simulink library "lib"  (R2021a)
settings: Solver=VariableStepAuto  StartTime=0.0  StopTime=10.0  RelTol=1e-3
values from neighbouring files (symbols this model uses):
  I = [I_x;I_y;I_z]    [DATA.m]
  I_inv = inv(I_matrix)    [DATA.m]
  I_matrix = diag(I)    [DATA.m]
  I_x = 91.6*1e-2    (= 0.916)    [DATA.m]
  I_y = 25.1*1e-2    (= 0.251)    [DATA.m]
  I_z = 100.9*1e-2    (= 1.009)    [DATA.m]
  om0 = deg2rad([10, -15, 5]')    [DATA.m]
  phi0_312 = -atan(A_313_0(2,1)/A_313_0(2,2))    [DATA.m]
  phi0_313 = deg2rad(9.7)    [DATA.m]
  psi0_312 = -atan(A_313_0(1,3)/A_313_0(3,3))    [DATA.m]
  psi0_313 = deg2rad(6)    [DATA.m]
  th0_312 = asin(A_313_0(2,3))    [DATA.m]
  th0_313 = deg2rad(19)    [DATA.m]
undefined symbols (not defined in the file or in its folder): dcm0, e, i, I_f, I_r, om0_f, om0_r, om0_x, om0_y, om0_z, orbit
libraries: $bdroot x8, vrlib x1
settings Model: Creator=dvd33  LastModifiedBy=dvd33
settings SolverCC: AlgebraicLoopSolver=TrustRegion
settings DebuggingCC: SFMachineParentedDataDiag=warning

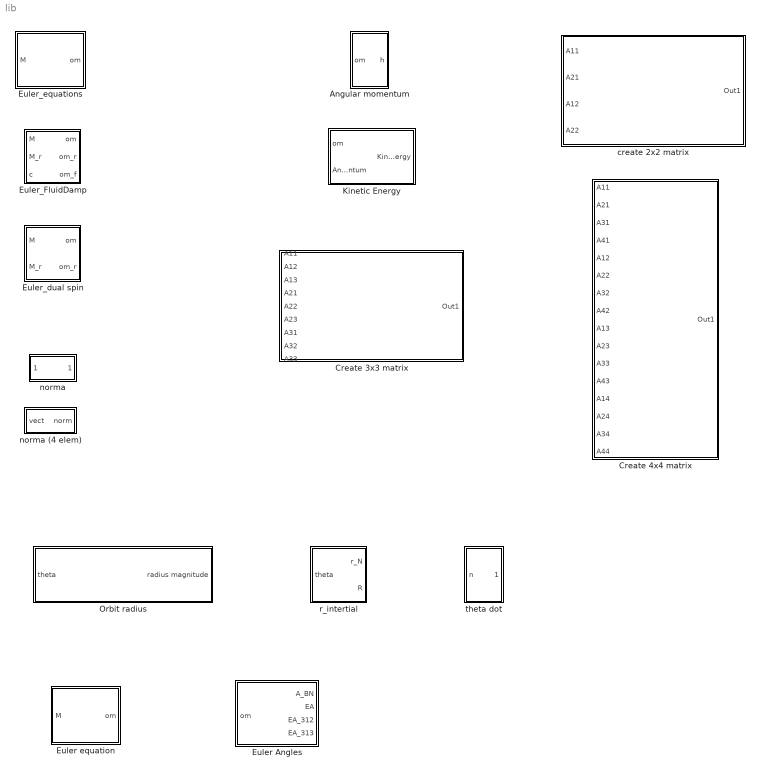
== system lib ==
  Angular momentum : Subsystem
  Create 3x3 matrix : Subsystem
  Create 4x4 matrix : Subsystem
  Euler Angles : Subsystem
  Euler equation : Subsystem
  Euler_FluidDamp : Subsystem
  Euler_dual spin : Subsystem
  Euler_equations : Subsystem
  Kinetic Energy : Subsystem
  Orbit radius : Subsystem
  create 2x2 matrix : Subsystem
  norma : Subsystem
  norma (4 elem) : Subsystem
  r_intertial : Subsystem
  theta dot : Subsystem

== system lib/Angular momentum ==
  om : Inport
  Demux : Demux  Outputs=3
  Gain : Gain  Gain=I_x
  Gain1 : Gain  Gain=I_y
  Gain2 : Gain  Gain=I_z
  Mux : Mux  Inputs=3
  h : Outport
  wires:
  Gain/1 -> Mux/1
  Demux/2 -> Gain1/1
  Gain1/1 -> Mux/2
  om/1 -> Demux/1
  Demux/3 -> Gain2/1
  Demux/1 -> Gain/1
  Mux/1 -> h/1  "Angular momentum"
  Gain2/1 -> Mux/3

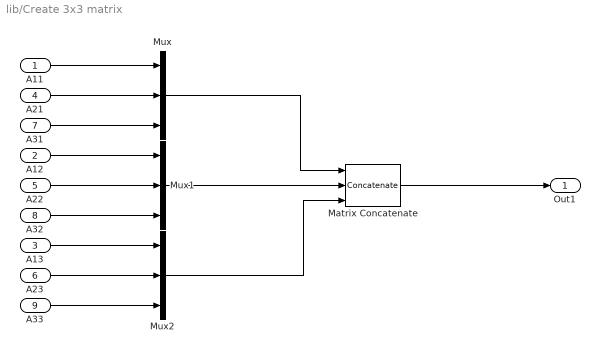
== system lib/Create 3x3 matrix ==
  A11 : Inport
  A12 : Inport  Port=2
  A13 : Inport  Port=3
  A21 : Inport  Port=4
  A22 : Inport  Port=5
  A23 : Inport  Port=6
  A31 : Inport  Port=7
  A32 : Inport  Port=8
  A33 : Inport  Port=9
  Matrix Concatenate : Concatenate  NumInputs=3  Mode=Multidimensional array  ConcatenateDimension=2
  Mux : Mux  Inputs=3
  Mux1 : Mux  Inputs=3
  Mux2 : Mux  Inputs=3
  Out1 : Outport
  wires:
  A33/1 -> Mux2/3
  A23/1 -> Mux2/2
  A13/1 -> Mux2/1
  A32/1 -> Mux1/3
  A22/1 -> Mux1/2
  A12/1 -> Mux1/1
  A21/1 -> Mux/2
  A31/1 -> Mux/3
  A11/1 -> Mux/1
  Mux2/1 -> Matrix Concatenate/3
  Mux1/1 -> Matrix Concatenate/2
  Mux/1 -> Matrix Concatenate/1
  Matrix Concatenate/1 -> Out1/1

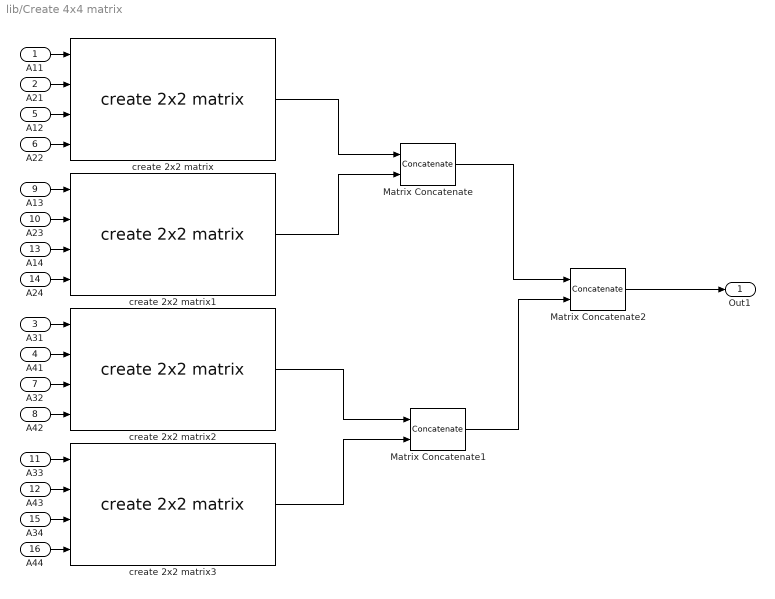
== system lib/Create 4x4 matrix ==
  A11 : Inport
  A21 : Inport  Port=2
  A31 : Inport  Port=3
  A41 : Inport  Port=4
  A12 : Inport  Port=5
  A22 : Inport  Port=6
  A32 : Inport  Port=7
  A42 : Inport  Port=8
  A13 : Inport  Port=9
  A23 : Inport  Port=10
  A33 : Inport  Port=11
  A43 : Inport  Port=12
  A14 : Inport  Port=13
  A24 : Inport  Port=14
  A34 : Inport  Port=15
  A44 : Inport  Port=16
  Matrix Concatenate : Concatenate  Mode=Multidimensional array
  Matrix Concatenate1 : Concatenate  Mode=Multidimensional array
  Matrix Concatenate2 : Concatenate  Mode=Multidimensional array  ConcatenateDimension=2
  create 2x2 matrix{,1..3} (4 alike) : $bdroot/create 2x2 matrix  SystemSampleTime=-1  Latency=0  AutoFrameSizeCalculation=off
  Out1 : Outport
  wires:
  A24/1 -> create 2x2 matrix1/4
  Matrix Concatenate1/1 -> Matrix Concatenate2/2
  create 2x2 matrix1/1 -> Matrix Concatenate/2
  Matrix Concatenate/1 -> Matrix Concatenate2/1
  create 2x2 matrix/1 -> Matrix Concatenate/1
  create 2x2 matrix2/1 -> Matrix Concatenate1/1
  A14/1 -> create 2x2 matrix1/3
  create 2x2 matrix3/1 -> Matrix Concatenate1/2
  A43/1 -> create 2x2 matrix3/2
  Matrix Concatenate2/1 -> Out1/1
  A34/1 -> create 2x2 matrix3/3
  A33/1 -> create 2x2 matrix3/1
  A44/1 -> create 2x2 matrix3/4
  A23/1 -> create 2x2 matrix1/2
  A32/1 -> create 2x2 matrix2/3
  A13/1 -> create 2x2 matrix1/1
  A21/1 -> create 2x2 matrix/2
  A12/1 -> create 2x2 matrix/3
  A42/1 -> create 2x2 matrix2/4
  A22/1 -> create 2x2 matrix/4
  A31/1 -> create 2x2 matrix2/1
  A11/1 -> create 2x2 matrix/1
  A41/1 -> create 2x2 matrix2/2

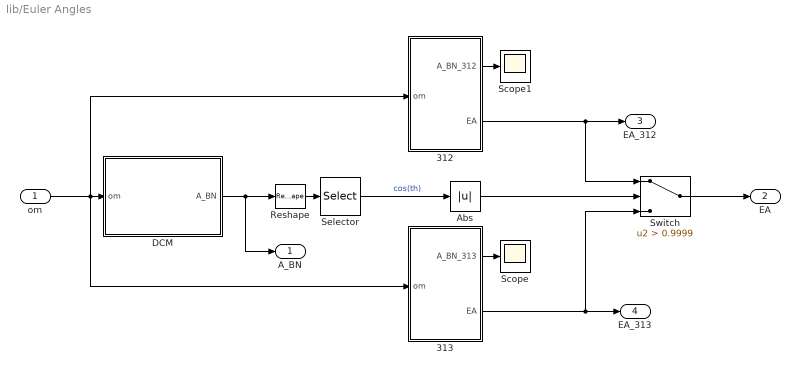
== system lib/Euler Angles ==
  om : Inport
  312 : Subsystem  TreatAsAtomicUnit=on
  313 : Subsystem  TreatAsAtomicUnit=on
  Abs : Abs
  DCM : Subsystem
  Reshape : Reshape
  Scope : Scope
  Scope1 : Scope
  Selector : Selector  InputPortWidth=9  IndexOptions=Index vector (dialog)  Indices=[9]  OutputSizes=1
  Switch : Switch  Criteria=u2 > Threshold  Threshold=0.9999
  A_BN : Outport
  EA : Outport  Port=2
  EA_312 : Outport  Port=3
  EA_313 : Outport  Port=4
  wires:
  om/1 -> 312/1(om), 313/1(om), DCM/1(om)
  DCM/1(A_BN) -> A_BN/1, Reshape/1
  Reshape/1 -> Selector/1
  Selector/1 -> Abs/1  "cos(th)"
  Abs/1 -> Switch/2
  313/1(A_BN_313) -> Scope/1
  312/1(A_BN_312) -> Scope1/1
  312/2(EA) -> EA_312/1, Switch/1
  313/2(EA) -> EA_313/1, Switch/3
  Switch/1 -> EA/1

== system lib/Euler equation ==
  M : Inport
  Cross Product : vrlib/Utilities/Cross Product
  Gain : Gain  Gain=I_matrix  Multiplication=Matrix(K*u) (u vector)
  Gain1 : Gain  Gain=I_inv  Multiplication=Matrix(K*u) (u vector)
  Integrator : Integrator  InitialCondition=om0
  Sum : Sum
  om : Outport
  wires:
  Gain/1 -> Cross Product/1
  Cross Product/1 -> Sum/1
  M/1 -> Sum/2
  Sum/1 -> Gain1/1
  Gain1/1 -> Integrator/1
  Integrator/1 -> Gain/1, Cross Product/2, om/1

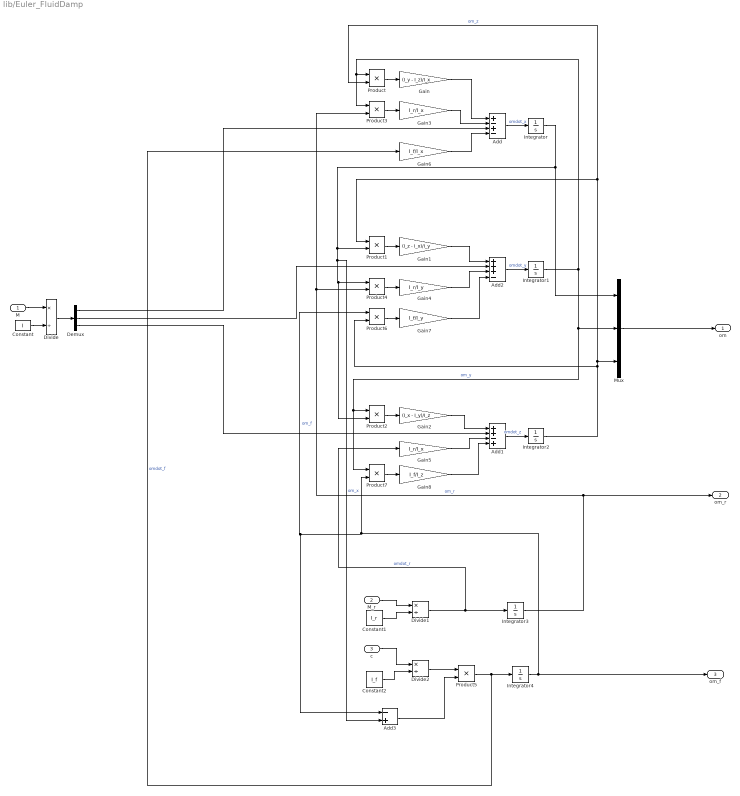
== system lib/Euler_FluidDamp ==
  M : Inport
  M_r : Inport  Port=2
  c : Inport  Port=3
  Add : Sum  Inputs=+-+-
  Add1 : Sum  Inputs=++-+
  Add2 : Sum  Inputs=+++-
  Add3 : Sum  Inputs=-+
  Constant : Constant  Value=I
  Constant1 : Constant  Value=I_r
  Constant2 : Constant  Value=I_f
  Demux : Demux  Outputs=3
  Divide : Product  Inputs=*/
  Divide1 : Product  Inputs=*/
  Divide2 : Product  Inputs=*/
  Gain : Gain  Gain=(I_y - I_z)/I_x
  Gain1 : Gain  Gain=(I_z - I_x)/I_y
  Gain2 : Gain  Gain=(I_x - I_y)/I_z
  Gain3 : Gain  Gain=I_r/I_x
  Gain4 : Gain  Gain=I_r/I_y
  Gain5 : Gain  Gain=I_r/I_x
  Gain6 : Gain  Gain=I_f/I_x
  Gain7 : Gain  Gain=I_f/I_y
  Gain8 : Gain  Gain=I_f/I_z
  Integrator : Integrator  InitialCondition=om0_x
  Integrator1 : Integrator  InitialCondition=om0_y
  Integrator2 : Integrator  InitialCondition=om0_z
  Integrator3 : Integrator  InitialCondition=om0_r
  Integrator4 : Integrator  InitialCondition=om0_f
  Mux : Mux  Inputs=3
  Product{,1..7} (8 alike) : Product
  om : Outport
  om_r : Outport  Port=2
  om_f : Outport  Port=3
  wires:
  Add3/1 -> Product5/2
  M/1 -> Divide/1
  Product5/1 -> Gain6/1, Integrator4/1  "omdot_f"
  Add/1 -> Integrator/1  "omdot_x"
  Integrator1/1 -> Product2/1, Product7/1, Mux/2, Product3/1, Product/1  "om_y"
  Integrator2/1 -> Product1/1, Product/2, Mux/3, Product6/2  "om_z"
  Product/1 -> Gain/1
  Add2/1 -> Integrator1/1  "omdot_y"
  Demux/3 -> Add1/2
  M_r/1 -> Divide1/1
  Product2/1 -> Gain2/1
  Gain7/1 -> Add2/4
  Gain8/1 -> Add1/4
  Integrator3/1 -> om_r/1, Product4/2, Product3/2  "om_r"
  Gain4/1 -> Add2/3
  Constant/1 -> Divide/2
  Product1/1 -> Gain1/1
  Integrator/1 -> Mux/1, Product2/2, Product4/1, Add3/2, Product1/2  "om_x"
  Gain1/1 -> Add2/1
  Demux/1 -> Add/3
  Constant2/1 -> Divide2/2
  Add1/1 -> Integrator2/1  "omdot_z"
  Product4/1 -> Gain4/1
  Demux/2 -> Add2/2
  c/1 -> Divide2/1
  Gain2/1 -> Add1/1
  Product6/1 -> Gain7/1
  Divide1/1 -> Gain5/1, Integrator3/1  "omdot_r"
  Divide2/1 -> Product5/1
  Gain5/1 -> Add1/3
  Product3/1 -> Gain3/1
  Constant1/1 -> Divide1/2
  Integrator4/1 -> om_f/1, Add3/1, Product6/1, Product7/2  "om_f"
  Gain6/1 -> Add/4
  Divide/1 -> Demux/1
  Gain/1 -> Add/1
  Product7/1 -> Gain8/1
  Gain3/1 -> Add/2
  Mux/1 -> om/1

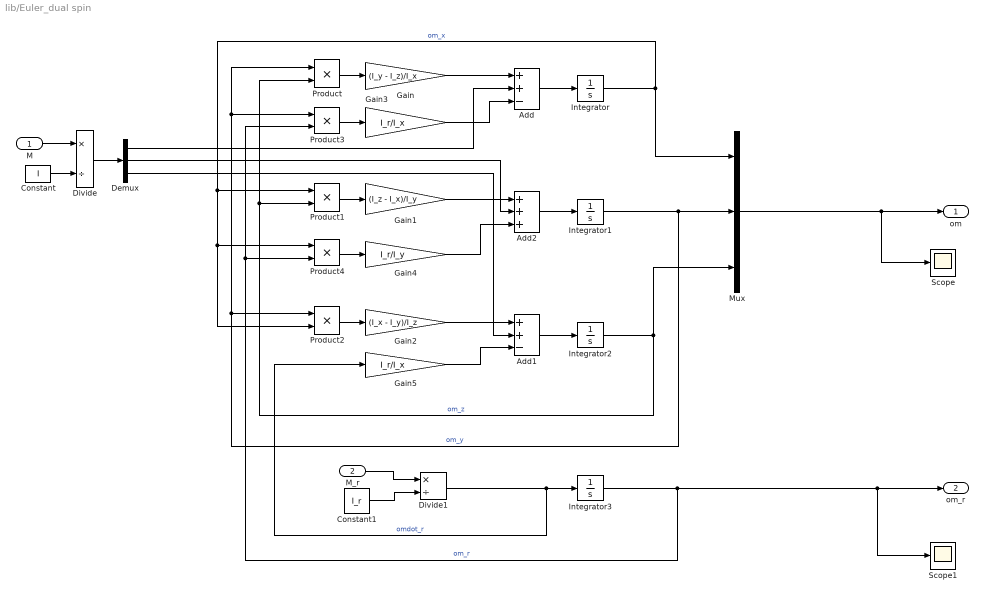
== system lib/Euler_dual spin ==
  M : Inport
  M_r : Inport  Port=2
  Add : Sum  Inputs=++-
  Add1 : Sum  Inputs=++-
  Add2 : Sum  Inputs=+++
  Constant : Constant  Value=I
  Constant1 : Constant  Value=I_r
  Demux : Demux  Outputs=3
  Divide : Product  Inputs=*/
  Divide1 : Product  Inputs=*/
  Gain : Gain  Gain=(I_y - I_z)/I_x
  Gain1 : Gain  Gain=(I_z - I_x)/I_y
  Gain2 : Gain  Gain=(I_x - I_y)/I_z
  Gain3 : Gain  Gain=I_r/I_x
  Gain4 : Gain  Gain=I_r/I_y
  Gain5 : Gain  Gain=I_r/I_x
  Integrator : Integrator  InitialCondition=om0_x
  Integrator1 : Integrator  InitialCondition=om0_y
  Integrator2 : Integrator  InitialCondition=om0_z
  Integrator3 : Integrator  InitialCondition=om0_r
  Mux : Mux  Inputs=3
  Product{,1..4} (5 alike) : Product
  Scope : Scope
  Scope1 : Scope
  om : Outport
  om_r : Outport  Port=2
  wires:
  Add2/1 -> Integrator1/1
  M_r/1 -> Divide1/1
  Product4/1 -> Gain4/1
  Gain5/1 -> Add1/3
  Demux/1 -> Add/2
  Product3/1 -> Gain3/1
  Add1/1 -> Integrator2/1
  Gain3/1 -> Add/3
  Add/1 -> Integrator/1
  Demux/3 -> Add1/2
  Integrator3/1 -> Scope1/1, om_r/1, Product3/2, Product4/2  "om_r"
  Constant1/1 -> Divide1/2
  Divide/1 -> Demux/1
  M/1 -> Divide/1
  Product2/1 -> Gain2/1
  Product/1 -> Gain/1
  Demux/2 -> Add2/2
  Divide1/1 -> Integrator3/1, Gain5/1  "omdot_r"
  Gain1/1 -> Add2/1
  Integrator/1 -> Product1/1, Product4/1, Product2/2, Mux/1  "om_x"
  Integrator2/1 -> Product/2, Product1/2, Mux/3  "om_z"
  Gain4/1 -> Add2/3
  Constant/1 -> Divide/2
  Integrator1/1 -> Mux/2, Product2/1, Product3/1, Product/1  "om_y"
  Gain/1 -> Add/1
  Gain2/1 -> Add1/1
  Product1/1 -> Gain1/1
  Mux/1 -> Scope/1, om/1

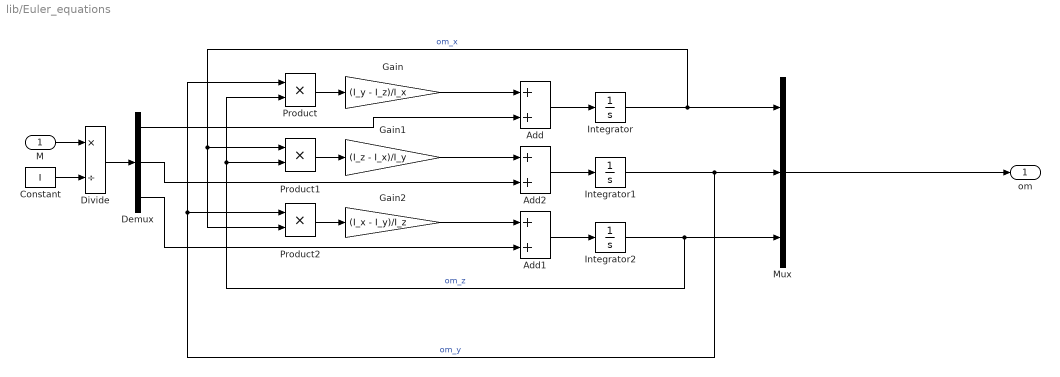
== system lib/Euler_equations ==
  M : Inport
  Add : Sum
  Add1 : Sum
  Add2 : Sum
  Constant : Constant  Value=I
  Demux : Demux  Outputs=3
  Divide : Product  Inputs=*/
  Gain : Gain  Gain=(I_y - I_z)/I_x
  Gain1 : Gain  Gain=(I_z - I_x)/I_y
  Gain2 : Gain  Gain=(I_x - I_y)/I_z
  Integrator : Integrator  InitialCondition=om0_x
  Integrator1 : Integrator  InitialCondition=om0_y
  Integrator2 : Integrator  InitialCondition=om0_z
  Mux : Mux  Inputs=3
  Product : Product
  Product1 : Product
  Product2 : Product
  om : Outport
  wires:
  Divide/1 -> Demux/1
  Product/1 -> Gain/1
  Demux/2 -> Add2/2
  Demux/1 -> Add/2
  Mux/1 -> om/1
  Gain1/1 -> Add2/1
  Gain/1 -> Add/1
  Constant/1 -> Divide/2
  Add/1 -> Integrator/1
  Demux/3 -> Add1/2
  Integrator1/1 -> Mux/2, Product/1, Product2/1  "om_y"
  Integrator/1 -> Mux/1, Product2/2, Product1/1  "om_x"
  Product1/1 -> Gain1/1
  Add2/1 -> Integrator1/1
  M/1 -> Divide/1
  Add1/1 -> Integrator2/1
  Product2/1 -> Gain2/1
  Gain2/1 -> Add1/1
  Integrator2/1 -> Mux/3, Product/2, Product1/2  "om_z"

== system lib/Kinetic Energy ==
  om : Inport
  Angular momentum : Inport  Port=2
  Dot Product : DotProduct  InputSameDT=on  OutDataTypeStr=Inherit: Inherit via internal rule
  Gain3 : Gain  Gain=0.5
  Kinectic Energy : Outport
  wires:
  Gain3/1 -> Dot Product/2
  om/1 -> Dot Product/1
  Dot Product/1 -> Kinectic Energy/1  "Kinectic Energy"
  Angular momentum/1 -> Gain3/1

== system lib/Orbit radius ==
  theta : Inport
  Add1 : Sum
  Constant : Constant  Value=orbit.a*(1-orbit.e^2)
  Constant1 : Constant
  Divide : Product  Inputs=*/
  Product : Product
  Trigonometric Function : Trigonometry  Operator=cos
  eccentricity : Constant  Value=orbit.e
  radius magnitude : Outport
  wires:
  Constant1/1 -> Add1/1
  theta/1 -> Trigonometric Function/1
  Trigonometric Function/1 -> Product/2
  Add1/1 -> Divide/2
  eccentricity/1 -> Product/1
  Divide/1 -> radius magnitude/1
  Product/1 -> Add1/2
  Constant/1 -> Divide/1

== system lib/create 2x2 matrix ==
  A11 : Inport
  A21 : Inport  Port=2
  A12 : Inport  Port=3
  A22 : Inport  Port=4
  Matrix Concatenate : Concatenate  Mode=Multidimensional array  ConcatenateDimension=2
  Mux : Mux  Inputs=2
  Mux1 : Mux  Inputs=2
  Out1 : Outport
  wires:
  Matrix Concatenate/1 -> Out1/1
  Mux/1 -> Matrix Concatenate/1
  Mux1/1 -> Matrix Concatenate/2
  A11/1 -> Mux/1
  A12/1 -> Mux/2
  A21/1 -> Mux1/1
  A22/1 -> Mux1/2

== system lib/norma ==
  vect : Inport
  Add : Sum  Inputs=+++
  Demux : Demux  Outputs=3
  Sqrt : Sqrt  SaturateOnIntegerOverflow=on
  Square : Math  Operator=square  SaturateOnIntegerOverflow=on
  Square1 : Math  Operator=square  SaturateOnIntegerOverflow=on
  Square2 : Math  Operator=square  SaturateOnIntegerOverflow=on
  norm : Outport
  wires:
  Add/1 -> Sqrt/1
  Square1/1 -> Add/2
  Square2/1 -> Add/3
  Sqrt/1 -> norm/1
  Demux/3 -> Square2/1
  Demux/2 -> Square1/1
  vect/1 -> Demux/1
  Square/1 -> Add/1
  Demux/1 -> Square/1

== system lib/norma (4 elem) ==
  vect : Inport
  Add : Sum  Inputs=++++
  Demux : Demux
  Sqrt : Sqrt  SaturateOnIntegerOverflow=on
  Square{,1..3} (4 alike) : Math  Operator=square  SaturateOnIntegerOverflow=on
  norm : Outport
  wires:
  vect/1 -> Demux/1
  Square/1 -> Add/1
  Demux/4 -> Square3/1
  Square2/1 -> Add/3
  Sqrt/1 -> norm/1
  Demux/1 -> Square/1
  Square1/1 -> Add/2
  Add/1 -> Sqrt/1
  Demux/2 -> Square1/1
  Demux/3 -> Square2/1
  Square3/1 -> Add/4

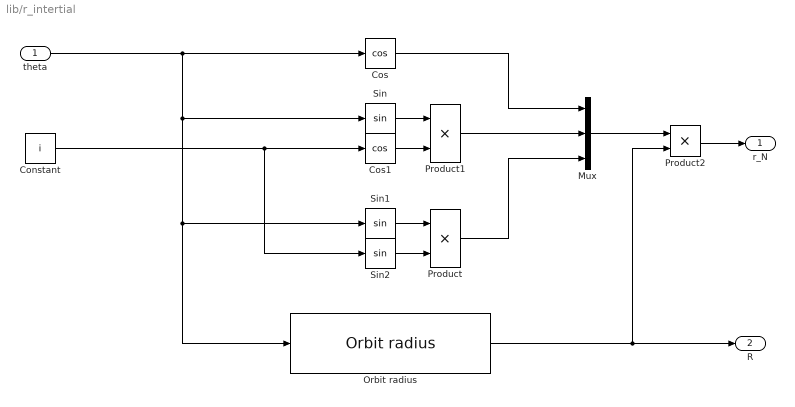
== system lib/r_intertial ==
  theta : Inport
  Constant : Constant  Value=i
  Cos : Trigonometry  Operator=cos
  Cos1 : Trigonometry  Operator=cos
  Mux : Mux  Inputs=3
  Orbit radius : $bdroot/Orbit radius  SystemSampleTime=-1  VariantActivationTime=update diagram  Latency=0  AutoFrameSizeCalculation=off
  Product : Product
  Product1 : Product
  Product2 : Product
  Sin : Trigonometry
  Sin1 : Trigonometry
  Sin2 : Trigonometry
  r_N : Outport
  R : Outport  Port=2
  wires:
  Mux/1 -> Product2/1
  Sin2/1 -> Product/2
  Orbit radius/1 -> R/1, Product2/2
  Cos/1 -> Mux/1
  Cos1/1 -> Product1/2
  Constant/1 -> Cos1/1, Sin2/1
  Product2/1 -> r_N/1
  Product/1 -> Mux/3
  theta/1 -> Sin1/1, Orbit radius/1, Sin/1, Cos/1
  Sin/1 -> Product1/1
  Product1/1 -> Mux/2
  Sin1/1 -> Product/1

== system lib/theta dot ==
  n : Inport
  Constant : Constant
  Constant1 : Constant  Value=(1-e^2)^(3/2)
  Cos : Trigonometry  Operator=cos
  Divide : Product  Inputs=*/
  Gain : Gain  Gain=e
  Integrator : Integrator
  Product : Product
  Square1 : Math  Operator=square  SaturateOnIntegerOverflow=on
  Sum1 : Sum
  theta : Outport
  wires:
  Divide/1 -> Integrator/1  "theta dot"
  Product/1 -> Divide/1
  Sum1/1 -> Square1/1
  Square1/1 -> Product/2
  Gain/1 -> Sum1/1
  Constant1/1 -> Divide/2
  Integrator/1 -> Cos/1, theta/1  "theta"
  Cos/1 -> Gain/1
  n/1 -> Product/1
  Constant/1 -> Sum1/2

== system lib/Euler Angles/312 ==
  om : Inport
  A_312 : Subsystem
  Angles 312 : Subsystem
  A_BN_312 : Outport
  EA : Outport  Port=2
  wires:
  A_312/1(A_BN_312) -> A_BN_312/1
  om/1 -> Angles 312/1(om)
  Angles 312/1(EA) -> EA/1, A_312/1(EA)

== system lib/Euler Angles/313 ==
  om : Inport
  A_313 : Subsystem
  Angles 313 : Subsystem
  Display : Display
  A_BN_313 : Outport
  EA : Outport  Port=2
  wires:
  om/1 -> Angles 313/1(om)
  A_313/1(A_BN_313) -> A_BN_313/1
  Angles 313/1(EA) -> Display/1, EA/1, A_313/1(EA)

== system lib/Euler Angles/DCM ==
  om : Inport
  Gain : Gain  Gain=-1
  Integrator : Integrator  InitialCondition=dcm0
  Matrix Multiply : Product  Multiplication=Matrix(*)
  Orthonormalization : Subsystem
  Subsystem : Subsystem
  A_BN : Outport
  wires:
  om/1 -> Subsystem/1(om)
  Subsystem/1(om^) -> Gain/1
  Gain/1 -> Matrix Multiply/1
  Matrix Multiply/1 -> Integrator/1
  Integrator/1 -> Orthonormalization/1(A0)
  Orthonormalization/1(A) -> A_BN/1, Matrix Multiply/2

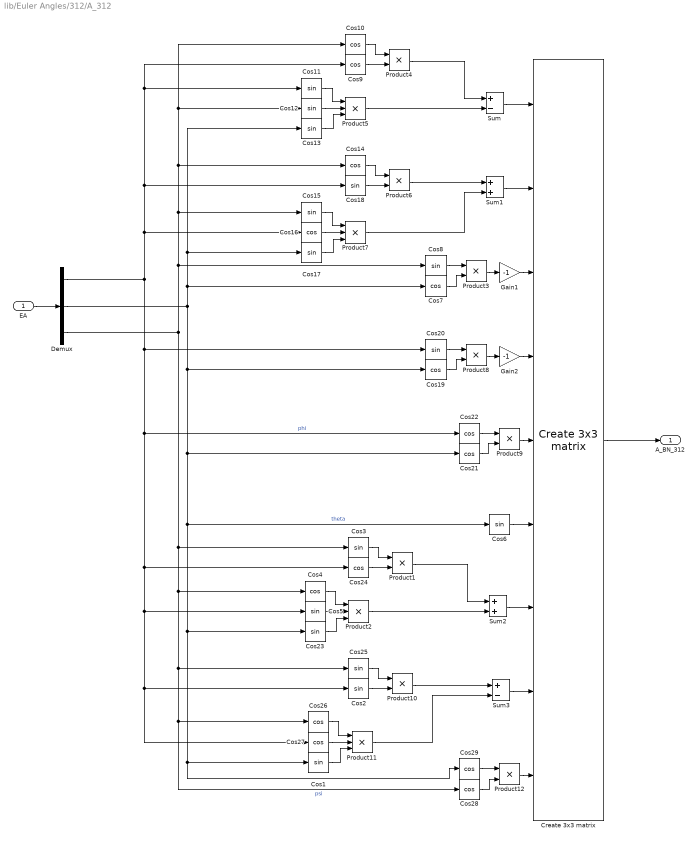
== system lib/Euler Angles/312/A_312 ==
  EA : Inport
  Cos{1..3,5..6,8,11..13,15,17..18,20,23,25} (15 alike) : Trigonometry
  Cos{4,7,9..10,14,16,19,21..22,24,26..29} (14 alike) : Trigonometry  Operator=cos
  Create 3x3 matrix : $bdroot/Create 3x3 matrix  SystemSampleTime=-1  VariantActivationTime=update diagram  Latency=0  AutoFrameSizeCalculation=off
  Demux : Demux  Outputs=3
  Gain1 : Gain  Gain=-1
  Gain2 : Gain  Gain=-1
  Product{1,3..4,6,8..10,12} (8 alike) : Product
  Product{2,5,7,11} (4 alike) : Product  Inputs=3
  Sum : Sum  Inputs=+-
  Sum1 : Sum
  Sum2 : Sum
  Sum3 : Sum  Inputs=+-
  A_BN_312 : Outport
  wires:
  Cos10/1 -> Product4/1
  Cos18/1 -> Product6/2
  Cos15/1 -> Product7/1
  Cos16/1 -> Product7/2
  Product3/1 -> Gain1/1
  Product7/1 -> Sum1/2
  Cos13/1 -> Product5/3
  Cos6/1 -> Create 3x3 matrix/6
  Cos14/1 -> Product6/1
  Cos17/1 -> Product7/3
  Cos11/1 -> Product5/1
  Product5/1 -> Sum/2
  Cos12/1 -> Product5/2
  Product4/1 -> Sum/1
  Sum1/1 -> Create 3x3 matrix/2
  Cos9/1 -> Product4/2
  Gain2/1 -> Create 3x3 matrix/4
  Cos8/1 -> Product3/1
  Cos7/1 -> Product3/2
  Sum/1 -> Create 3x3 matrix/1
  Product6/1 -> Sum1/1
  Create 3x3 matrix/1 -> A_BN_312/1
  Gain1/1 -> Create 3x3 matrix/3
  Cos19/1 -> Product8/2
  Cos20/1 -> Product8/1
  Product8/1 -> Gain2/1
  Cos21/1 -> Product9/2
  Cos22/1 -> Product9/1
  Product9/1 -> Create 3x3 matrix/5
  Sum2/1 -> Create 3x3 matrix/7
  Cos3/1 -> Product1/1
  Product1/1 -> Sum2/1
  Cos24/1 -> Product1/2
  Cos5/1 -> Product2/2
  Product2/1 -> Sum2/2
  Cos4/1 -> Product2/1
  Cos23/1 -> Product2/3
  Cos1/1 -> Product11/3
  Cos26/1 -> Product11/1
  Cos2/1 -> Product10/2
  Product10/1 -> Sum3/1
  Cos25/1 -> Product10/1
  Product11/1 -> Sum3/2
  Cos27/1 -> Product11/2
  Sum3/1 -> Create 3x3 matrix/8
  Cos28/1 -> Product12/2
  Cos29/1 -> Product12/1
  Product12/1 -> Create 3x3 matrix/9
  Demux/2 -> Cos17/1, Cos13/1, Cos7/1, Cos19/1, Cos21/1, Cos6/1, Cos23/1, Cos29/1, Cos1/1  "theta"
  Demux/3 -> Cos28/1, Cos26/1, Cos25/1, Cos4/1, Cos3/1, Cos12/1, Cos10/1, Cos14/1, Cos15/1, Cos8/1  "psi"
  Demux/1 -> Cos11/1, Cos9/1, Cos18/1, Cos16/1, Cos20/1, Cos22/1, Cos2/1, Cos27/1, Cos5/1, Cos24/1  "phi"
  EA/1 -> Demux/1

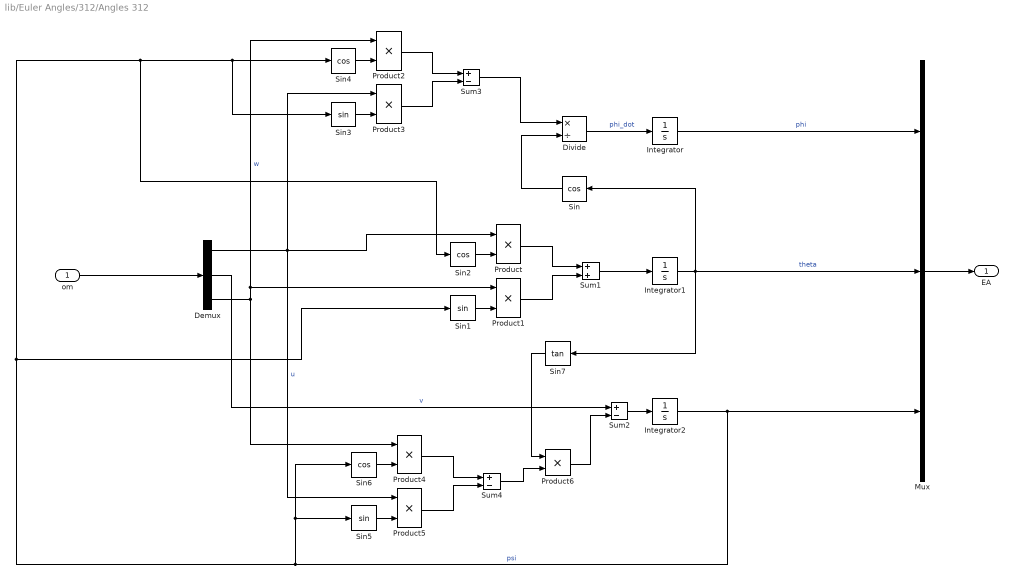
== system lib/Euler Angles/312/Angles 312 ==
  om : Inport
  Demux : Demux  Outputs=3
  Divide : Product  Inputs=*/
  Integrator : Integrator  InitialCondition=phi0_312  WrapState=on
  Integrator1 : Integrator  InitialCondition=th0_312  WrapState=on
  Integrator2 : Integrator  InitialCondition=psi0_312  WrapState=on
  Mux : Mux  Inputs=3
  Product{,1..6} (7 alike) : Product
  Sin{,2,4,6} (4 alike) : Trigonometry  Operator=cos
  Sin1 : Trigonometry
  Sin3 : Trigonometry
  Sin5 : Trigonometry
  Sin7 : Trigonometry  Operator=tan
  Sum1 : Sum
  Sum2 : Sum  Inputs=+-
  Sum3 : Sum  Inputs=+-
  Sum4 : Sum  Inputs=+-
  EA : Outport
  wires:
  Sin2/1 -> Product/2
  Sum2/1 -> Integrator2/1
  Product2/1 -> Sum3/1
  Sin7/1 -> Product6/1
  Product/1 -> Sum1/1
  Sin/1 -> Divide/2
  Demux/1 -> Product5/1, Product/1, Product3/1  "u"
  Product3/1 -> Sum3/2
  Integrator/1 -> Mux/1  "phi"
  Integrator1/1 -> Sin7/1, Mux/2, Sin/1  "theta"
  Sin6/1 -> Product4/2
  Product5/1 -> Sum4/2
  Sum3/1 -> Divide/1
  Product4/1 -> Sum4/1
  om/1 -> Demux/1
  Sin5/1 -> Product5/2
  Product6/1 -> Sum2/2
  Sum1/1 -> Integrator1/1
  Divide/1 -> Integrator/1  "phi_dot"
  Sin3/1 -> Product3/2
  Sin1/1 -> Product1/2
  Product1/1 -> Sum1/2
  Sin4/1 -> Product2/2
  Demux/3 -> Product4/1, Product1/1, Product2/1  "w"
  Integrator2/1 -> Sin1/1, Sin2/1, Sin4/1, Sin3/1, Sin5/1, Sin6/1, Mux/3  "psi"
  Demux/2 -> Sum2/1  "v"
  Sum4/1 -> Product6/2
  Mux/1 -> EA/1

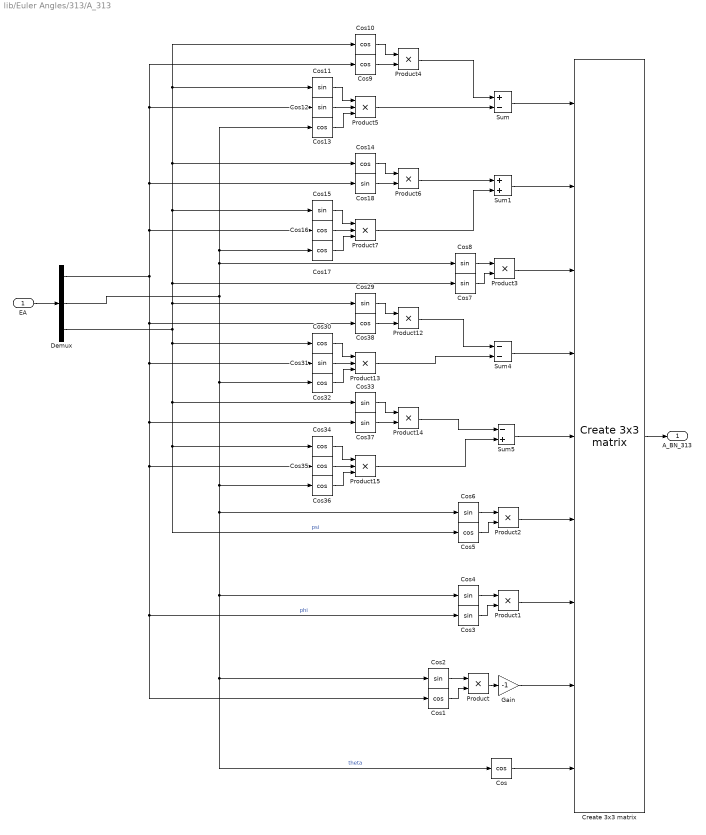
== system lib/Euler Angles/313/A_313 ==
  EA : Inport
  Cos{,1,5,9..10,13..14,16..17,30,32,34..36,38} (15 alike) : Trigonometry  Operator=cos
  Cos{2..4,6..8,11..12,15,18,29,31,33,37} (14 alike) : Trigonometry
  Create 3x3 matrix : $bdroot/Create 3x3 matrix  SystemSampleTime=-1  VariantActivationTime=update diagram  Latency=0  AutoFrameSizeCalculation=off
  Demux : Demux  Outputs=3
  Gain : Gain  Gain=-1
  Product{,1..4,6,12,14} (8 alike) : Product
  Product{5,7,13,15} (4 alike) : Product  Inputs=3
  Sum : Sum  Inputs=+-
  Sum1 : Sum
  Sum4 : Sum  Inputs=--
  Sum5 : Sum  Inputs=-+
  A_BN_313 : Outport
  wires:
  Cos1/1 -> Product/2
  Cos30/1 -> Product13/1
  Cos35/1 -> Product15/2
  Product1/1 -> Create 3x3 matrix/7
  Create 3x3 matrix/1 -> A_BN_313/1
  Product6/1 -> Sum1/1
  Cos/1 -> Create 3x3 matrix/9
  Cos31/1 -> Product13/2
  Cos34/1 -> Product15/1
  Product13/1 -> Sum4/2
  Sum/1 -> Create 3x3 matrix/1
  Cos7/1 -> Product3/2
  Cos32/1 -> Product13/3
  Cos8/1 -> Product3/1
  Sum4/1 -> Create 3x3 matrix/4
  Gain/1 -> Create 3x3 matrix/8
  Sum5/1 -> Create 3x3 matrix/5
  Cos9/1 -> Product4/2
  Sum1/1 -> Create 3x3 matrix/2
  Cos3/1 -> Product1/2
  Product4/1 -> Sum/1
  Cos2/1 -> Product/1
  Cos12/1 -> Product5/2
  Product5/1 -> Sum/2
  Product12/1 -> Sum4/1
  Cos33/1 -> Product14/1
  Cos11/1 -> Product5/1
  Cos29/1 -> Product12/1
  Cos17/1 -> Product7/3
  Product/1 -> Gain/1
  Cos37/1 -> Product14/2
  Product14/1 -> Sum5/1
  Product2/1 -> Create 3x3 matrix/6
  Cos14/1 -> Product6/1
  Cos6/1 -> Product2/1
  Cos4/1 -> Product1/1
  Cos13/1 -> Product5/3
  Product7/1 -> Sum1/2
  Product3/1 -> Create 3x3 matrix/3
  Cos38/1 -> Product12/2
  Demux/3 -> Cos33/1, Cos34/1, Cos5/1, Cos30/1, Cos11/1, Cos10/1, Cos14/1, Cos15/1, Cos7/1, Cos29/1  "psi"
  Cos5/1 -> Product2/2
  Cos16/1 -> Product7/2
  Cos36/1 -> Product15/3
  Cos15/1 -> Product7/1
  Demux/1 -> Cos16/1, Cos18/1, Cos12/1, Cos9/1, Cos31/1, Cos35/1, Cos1/1, Cos3/1, Cos37/1, Cos38/1  "phi"
  Cos18/1 -> Product6/2
  Product15/1 -> Sum5/2
  Demux/2 -> Cos13/1, Cos17/1, Cos8/1, Cos36/1, Cos2/1, Cos/1, Cos4/1, Cos6/1, Cos32/1  "theta"
  Cos10/1 -> Product4/1
  EA/1 -> Demux/1

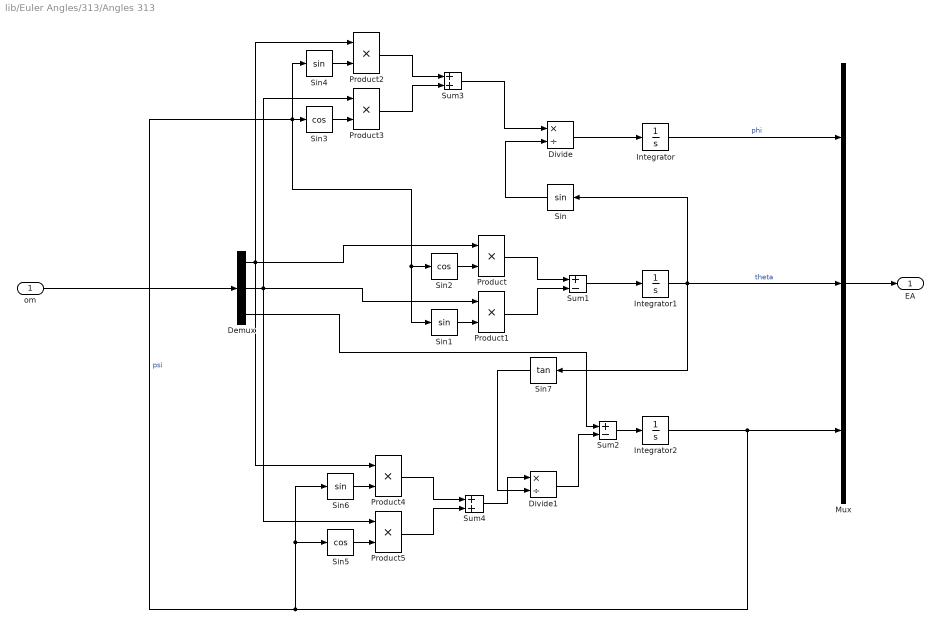
== system lib/Euler Angles/313/Angles 313 ==
  om : Inport
  Demux : Demux  Outputs=3
  Divide : Product  Inputs=*/
  Divide1 : Product  Inputs=*/
  Integrator : Integrator  InitialCondition=phi0_313  WrapState=on
  Integrator1 : Integrator  InitialCondition=th0_313  WrapState=on
  Integrator2 : Integrator  InitialCondition=psi0_313  WrapState=on
  Mux : Mux  Inputs=3
  Product{,1..5} (6 alike) : Product
  Sin{,1,4,6} (4 alike) : Trigonometry
  Sin2 : Trigonometry  Operator=cos
  Sin3 : Trigonometry  Operator=cos
  Sin5 : Trigonometry  Operator=cos
  Sin7 : Trigonometry  Operator=tan
  Sum1 : Sum  Inputs=+-
  Sum2 : Sum  Inputs=+-
  Sum3 : Sum
  Sum4 : Sum
  EA : Outport
  wires:
  Integrator2/1 -> Sin5/1, Sin6/1, Sin3/1, Sin4/1, Sin1/1, Sin2/1, Mux/3  "psi"
  Demux/3 -> Sum2/1
  Sin4/1 -> Product2/2
  Product1/1 -> Sum1/2
  Sin1/1 -> Product1/2
  Sin3/1 -> Product3/2
  Demux/2 -> Product1/1, Product5/1, Product3/1
  Divide/1 -> Integrator/1
  Sum1/1 -> Integrator1/1
  Divide1/1 -> Sum2/2
  Sin5/1 -> Product5/2
  Sum4/1 -> Divide1/1
  om/1 -> Demux/1
  Product4/1 -> Sum4/1
  Sum3/1 -> Divide/1
  Product5/1 -> Sum4/2
  Sin6/1 -> Product4/2
  Integrator/1 -> Mux/1  "phi"
  Product3/1 -> Sum3/2
  Demux/1 -> Product4/1, Product2/1, Product/1
  Sin/1 -> Divide/2
  Product/1 -> Sum1/1
  Sin7/1 -> Divide1/2
  Product2/1 -> Sum3/1
  Sum2/1 -> Integrator2/1
  Sin2/1 -> Product/2
  Mux/1 -> EA/1
  Integrator1/1 -> Sin7/1, Mux/2, Sin/1  "theta"

== system lib/Euler Angles/DCM/Orthonormalization ==
  A0 : Inport
  Gain : Gain  Gain=3/2
  Gain1 : Gain  Gain=1/2
  Matrix Multiply : Product  Inputs=3  Multiplication=Matrix(*)
  Sum : Sum  Inputs=+-
  Transpose : Math  Operator=transpose  SaturateOnIntegerOverflow=on
  A : Outport
  wires:
  Sum/1 -> A/1
  Gain/1 -> Sum/1
  A0/1 -> Matrix Multiply/1, Transpose/1, Gain1/1, Gain/1
  Transpose/1 -> Matrix Multiply/2
  Gain1/1 -> Matrix Multiply/3
  Matrix Multiply/1 -> Sum/2

== system lib/Euler Angles/DCM/Subsystem ==
  om : Inport
  Constant : Constant  Value=0
  Create 3x3 matrix : $bdroot/Create 3x3 matrix  SystemSampleTime=-1  VariantActivationTime=update diagram  Latency=0  AutoFrameSizeCalculation=off
  Demux : Demux  Outputs=3
  Gain : Gain  Gain=-1
  Gain1 : Gain  Gain=-1
  Gain2 : Gain  Gain=-1
  om^ : Outport
  wires:
  Create 3x3 matrix/1 -> om^/1
  Constant/1 -> Create 3x3 matrix/9, Create 3x3 matrix/5, Create 3x3 matrix/1
  om/1 -> Demux/1
  Demux/1 -> Gain1/1, Create 3x3 matrix/8
  Demux/3 -> Create 3x3 matrix/4, Gain/1
  Demux/2 -> Gain2/1, Create 3x3 matrix/3
  Gain/1 -> Create 3x3 matrix/2
  Gain1/1 -> Create 3x3 matrix/6
  Gain2/1 -> Create 3x3 matrix/7
